simulink model "FFM_Punch"  (R2017a)
settings: Solver=ode3  StartTime=0.0  StopTime=timesteps  FixedStep=data.SIM.Ts  RelTol=1e-3  EnableMultiTasking=on
values from neighbouring files (symbols this model uses):
  data =     [dakota_config.mat]
  downshift_map = data.TCU.upshift.veh_spd_default    [Simulation_results.m]
  upshift_map = data.TCU.upshift.veh_spd_default    [Simulation_results.m]
undefined symbols (not defined in the file or in its folder): air_density, Cd, DiscIntNeverNeededParam, fr_crankshaft, fr_speed_values, g, i_FD, ICE, Low_Ratio, M_Eng_Max, M_Eng_Max_Max, M_Eng_Max_Rpm, mt2m_f, mu_Roll_C0, mu_Roll_C1, mu_Roll_C2, Mv, n_Idle_Eng, Overdrive_Ratio, Re, S_eff_drag, Ts
(part 5 of 15)

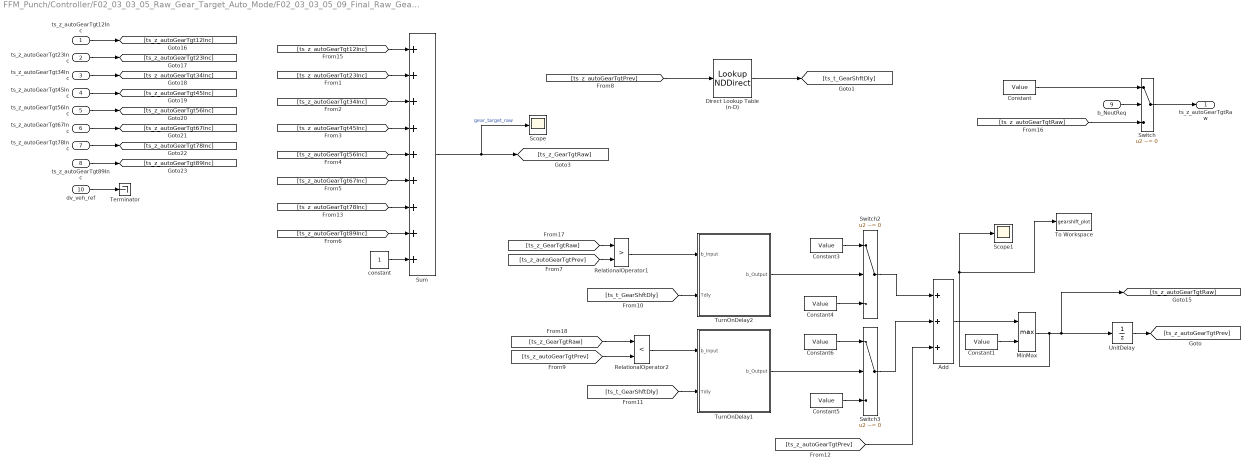
== system FFM_Punch/Controller/F02_03_03_05_Raw_Gear_Target_Auto_Mode/F02_03_03_05_09_Final_Raw_Gear_Target_Auto_Mode ==
  ts_z_autoGearTgt12Inc : Inport
  ts_z_autoGearTgt23Inc : Inport  Port=2
  ts_z_autoGearTgt34Inc : Inport  Port=3
  ts_z_autoGearTgt45Inc : Inport  Port=4
  ts_z_autoGearTgt56Inc : Inport  Port=5
  ts_z_autoGearTgt67Inc : Inport  Port=6
  ts_z_autoGearTgt78Inc : Inport  Port=7
  ts_z_autoGearTgt89Inc : Inport  Port=8
  b_NeutReq : Inport  Port=9
  dv_veh_ref : Inport  Tag=Controls_Lib  Description=Inp  Port=10  Interpolate=off
  Add : Sum  Inputs=+++
  Constant : Constant  Tag=Controls_Lib  Description=constant  Value=Value  OutMin=OutMin  OutMax=OutMax  OutDataTypeStr=int8  SampleTime=SampleTime  FramePeriod=FramePeriod  mask(Constant){Value=0, VectorParams1D=on, SampleTime=-1, FramePeriod=inf, OutMin=[], OutMax=[], OutDataTypeStr=int8, LockScale=off}
      mask prompts: Value "Simulink:blkprm_prompts:ConstConstValue"; VectorParams1D "Simulink:blkprm_prompts:AllSrcsVector1D"; SampleTime "Simulink:blkprm_prompts:AllSrcBlksSampleTime"; FramePeriod "Simulink:blkprm_prompts:AllSrcBlksFramePeriod"; OutMin "Simulink:blkprm_prompts:OutputDesignMin"; OutMax "Simulink:blkprm_prompts:OutputDesignMax"; OutDataTypeStr "Simulink:blkprm_prompts:OUTPUT_UNIFIEDDATATYPE"; LockScale "Simulink:blkprm_prompts:LockScale"
      mask help: Output the constant specified by the 'Constant value' parameter.
      mask Help: web([fileparts(which('Lib_built')) filesep 'hlp' filesep 'lib_constant' '.html'], '-helpbrowser')
      mask TypeOptions Value: Value
      mask TypeOptions VectorParams1D: VectorParams1D
      mask TypeOptions SampleTime: SampleTime
      mask TypeOptions FramePeriod: FramePeriod
      mask TypeOptions OutMin: OutMin
      mask TypeOptions OutMax: OutMax
      mask TypeOptions OutDataTypeStr: OutDataTypeStr
      mask TypeOptions LockScale: LockScale
      mask DialogControl ParameterTabVar0 Prompt: Main
      mask Display: disp(get_param(gcb,'Value'))
  Constant1 : Constant  Tag=Controls_Lib  Description=constant  Value=Value  OutMin=OutMin  OutMax=OutMax  OutDataTypeStr=int8  SampleTime=SampleTime  FramePeriod=FramePeriod  mask(Constant){Value=1, VectorParams1D=on, SampleTime=-1, FramePeriod=inf, OutMin=[], OutMax=[], OutDataTypeStr=int8, LockScale=off}
      mask prompts: Value "Simulink:blkprm_prompts:ConstConstValue"; VectorParams1D "Simulink:blkprm_prompts:AllSrcsVector1D"; SampleTime "Simulink:blkprm_prompts:AllSrcBlksSampleTime"; FramePeriod "Simulink:blkprm_prompts:AllSrcBlksFramePeriod"; OutMin "Simulink:blkprm_prompts:OutputDesignMin"; OutMax "Simulink:blkprm_prompts:OutputDesignMax"; OutDataTypeStr "Simulink:blkprm_prompts:OUTPUT_UNIFIEDDATATYPE"; LockScale "Simulink:blkprm_prompts:LockScale"
      mask help: Output the constant specified by the 'Constant value' parameter.
      mask Help: web([fileparts(which('Lib_built')) filesep 'hlp' filesep 'lib_constant' '.html'], '-helpbrowser')
      mask TypeOptions Value: Value
      mask TypeOptions VectorParams1D: VectorParams1D
      mask TypeOptions SampleTime: SampleTime
      mask TypeOptions FramePeriod: FramePeriod
      mask TypeOptions OutMin: OutMin
      mask TypeOptions OutMax: OutMax
      mask TypeOptions OutDataTypeStr: OutDataTypeStr
      mask TypeOptions LockScale: LockScale
      mask DialogControl ParameterTabVar0 Prompt: Main
      mask Display: disp(get_param(gcb,'Value'))
  Constant3 : Constant  Tag=Controls_Lib  Description=constant  Value=Value  OutMin=OutMin  OutMax=OutMax  OutDataTypeStr=int8  SampleTime=SampleTime  FramePeriod=FramePeriod  mask(Constant){Value=1, VectorParams1D=on, SampleTime=-1, FramePeriod=inf, OutMin=[], OutMax=[], OutDataTypeStr=int8, LockScale=off}
      mask prompts: Value "Simulink:blkprm_prompts:ConstConstValue"; VectorParams1D "Simulink:blkprm_prompts:AllSrcsVector1D"; SampleTime "Simulink:blkprm_prompts:AllSrcBlksSampleTime"; FramePeriod "Simulink:blkprm_prompts:AllSrcBlksFramePeriod"; OutMin "Simulink:blkprm_prompts:OutputDesignMin"; OutMax "Simulink:blkprm_prompts:OutputDesignMax"; OutDataTypeStr "Simulink:blkprm_prompts:OUTPUT_UNIFIEDDATATYPE"; LockScale "Simulink:blkprm_prompts:LockScale"
      mask help: Output the constant specified by the 'Constant value' parameter.
      mask Help: web([fileparts(which('Lib_built')) filesep 'hlp' filesep 'lib_constant' '.html'], '-helpbrowser')
      mask TypeOptions Value: Value
      mask TypeOptions VectorParams1D: VectorParams1D
      mask TypeOptions SampleTime: SampleTime
      mask TypeOptions FramePeriod: FramePeriod
      mask TypeOptions OutMin: OutMin
      mask TypeOptions OutMax: OutMax
      mask TypeOptions OutDataTypeStr: OutDataTypeStr
      mask TypeOptions LockScale: LockScale
      mask DialogControl ParameterTabVar0 Prompt: Main
      mask Display: disp(get_param(gcb,'Value'))
  Constant4 : Constant  Tag=Controls_Lib  Description=constant  Value=Value  OutMin=OutMin  OutMax=OutMax  OutDataTypeStr=int8  SampleTime=SampleTime  FramePeriod=FramePeriod  mask(Constant){Value=0, VectorParams1D=on, SampleTime=-1, FramePeriod=inf, OutMin=[], OutMax=[], OutDataTypeStr=int8, LockScale=off}
      mask prompts: Value "Simulink:blkprm_prompts:ConstConstValue"; VectorParams1D "Simulink:blkprm_prompts:AllSrcsVector1D"; SampleTime "Simulink:blkprm_prompts:AllSrcBlksSampleTime"; FramePeriod "Simulink:blkprm_prompts:AllSrcBlksFramePeriod"; OutMin "Simulink:blkprm_prompts:OutputDesignMin"; OutMax "Simulink:blkprm_prompts:OutputDesignMax"; OutDataTypeStr "Simulink:blkprm_prompts:OUTPUT_UNIFIEDDATATYPE"; LockScale "Simulink:blkprm_prompts:LockScale"
      mask help: Output the constant specified by the 'Constant value' parameter.
      mask Help: web([fileparts(which('Lib_built')) filesep 'hlp' filesep 'lib_constant' '.html'], '-helpbrowser')
      mask TypeOptions Value: Value
      mask TypeOptions VectorParams1D: VectorParams1D
      mask TypeOptions SampleTime: SampleTime
      mask TypeOptions FramePeriod: FramePeriod
      mask TypeOptions OutMin: OutMin
      mask TypeOptions OutMax: OutMax
      mask TypeOptions OutDataTypeStr: OutDataTypeStr
      mask TypeOptions LockScale: LockScale
      mask DialogControl ParameterTabVar0 Prompt: Main
      mask Display: disp(get_param(gcb,'Value'))
  Constant5 : Constant  Tag=Controls_Lib  Description=constant  Value=Value  OutMin=OutMin  OutMax=OutMax  OutDataTypeStr=int8  SampleTime=SampleTime  FramePeriod=FramePeriod  mask(Constant){Value=0, VectorParams1D=on, SampleTime=-1, FramePeriod=inf, OutMin=[], OutMax=[], OutDataTypeStr=int8, LockScale=off}
      mask prompts: Value "Simulink:blkprm_prompts:ConstConstValue"; VectorParams1D "Simulink:blkprm_prompts:AllSrcsVector1D"; SampleTime "Simulink:blkprm_prompts:AllSrcBlksSampleTime"; FramePeriod "Simulink:blkprm_prompts:AllSrcBlksFramePeriod"; OutMin "Simulink:blkprm_prompts:OutputDesignMin"; OutMax "Simulink:blkprm_prompts:OutputDesignMax"; OutDataTypeStr "Simulink:blkprm_prompts:OUTPUT_UNIFIEDDATATYPE"; LockScale "Simulink:blkprm_prompts:LockScale"
      mask help: Output the constant specified by the 'Constant value' parameter.
      mask Help: web([fileparts(which('Lib_built')) filesep 'hlp' filesep 'lib_constant' '.html'], '-helpbrowser')
      mask TypeOptions Value: Value
      mask TypeOptions VectorParams1D: VectorParams1D
      mask TypeOptions SampleTime: SampleTime
      mask TypeOptions FramePeriod: FramePeriod
      mask TypeOptions OutMin: OutMin
      mask TypeOptions OutMax: OutMax
      mask TypeOptions OutDataTypeStr: OutDataTypeStr
      mask TypeOptions LockScale: LockScale
      mask DialogControl ParameterTabVar0 Prompt: Main
      mask Display: disp(get_param(gcb,'Value'))
  Constant6 : Constant  Tag=Controls_Lib  Description=constant  Value=Value  OutMin=OutMin  OutMax=OutMax  OutDataTypeStr=int8  SampleTime=SampleTime  FramePeriod=FramePeriod  mask(Constant){Value=-1, VectorParams1D=on, SampleTime=-1, FramePeriod=inf, OutMin=[], OutMax=[], OutDataTypeStr=int8, LockScale=off}
      mask prompts: Value "Simulink:blkprm_prompts:ConstConstValue"; VectorParams1D "Simulink:blkprm_prompts:AllSrcsVector1D"; SampleTime "Simulink:blkprm_prompts:AllSrcBlksSampleTime"; FramePeriod "Simulink:blkprm_prompts:AllSrcBlksFramePeriod"; OutMin "Simulink:blkprm_prompts:OutputDesignMin"; OutMax "Simulink:blkprm_prompts:OutputDesignMax"; OutDataTypeStr "Simulink:blkprm_prompts:OUTPUT_UNIFIEDDATATYPE"; LockScale "Simulink:blkprm_prompts:LockScale"
      mask help: Output the constant specified by the 'Constant value' parameter.
      mask Help: web([fileparts(which('Lib_built')) filesep 'hlp' filesep 'lib_constant' '.html'], '-helpbrowser')
      mask TypeOptions Value: Value
      mask TypeOptions VectorParams1D: VectorParams1D
      mask TypeOptions SampleTime: SampleTime
      mask TypeOptions FramePeriod: FramePeriod
      mask TypeOptions OutMin: OutMin
      mask TypeOptions OutMax: OutMax
      mask TypeOptions OutDataTypeStr: OutDataTypeStr
      mask TypeOptions LockScale: LockScale
      mask DialogControl ParameterTabVar0 Prompt: Main
      mask Display: disp(get_param(gcb,'Value'))
  Direct Lookup Table (n-D) : LookupNDDirect  NumberOfTableDimensions=1  Table=data.TCU.gearShiftDelay  DiagnosticForOutOfRangeInput=None  TableDataTypeStr=single
  MinMax : MinMax  Function=max  Inputs=2
  RelationalOperator1 : RelationalOperator  Tag=Controls_Lib  Description=RelationalOperator  Operator=>  OutDataTypeStr=boolean  SampleTime=SampleTime  RndMeth=Nearest  InputSameDT=on  mask(Relational operator){Operator=>, ZeroCross=on, SampleTime=-1, InputSameDT=on, OutDataTypeStr=boolean}
      mask prompts: Operator "Relational operator:"; ZeroCross "Enable zero-crossing detection"; SampleTime "Sample time (-1 for inherited):"; InputSameDT "Require all inputs to have the same data type"; OutDataTypeStr "Output data type:"
      mask help: Applies the selected relational operator to the inputs and outputs the result. The top (or left) input corresponds to the first operand.
      mask Help: web([fileparts(which('Lib_built')) filesep 'hlp' filesep 'lib_Relational' '.html'], '-helpbrowser')
      mask TypeOptions Operator: Operator
      mask TypeOptions ZeroCross: ZeroCross
      mask TypeOptions SampleTime: SampleTime
      mask TypeOptions InputSameDT: InputSameDT
      mask TypeOptions OutDataTypeStr: OutDataTypeStr
  RelationalOperator2 : RelationalOperator  Tag=Controls_Lib  Description=RelationalOperator  Operator=<  OutDataTypeStr=boolean  SampleTime=SampleTime  RndMeth=Nearest  InputSameDT=on  mask(Relational operator){Operator=<, ZeroCross=on, SampleTime=-1, InputSameDT=on, OutDataTypeStr=boolean}
      mask prompts: Operator "Relational operator:"; ZeroCross "Enable zero-crossing detection"; SampleTime "Sample time (-1 for inherited):"; InputSameDT "Require all inputs to have the same data type"; OutDataTypeStr "Output data type:"
      mask help: Applies the selected relational operator to the inputs and outputs the result. The top (or left) input corresponds to the first operand.
      mask Help: web([fileparts(which('Lib_built')) filesep 'hlp' filesep 'lib_Relational' '.html'], '-helpbrowser')
      mask TypeOptions Operator: Operator
      mask TypeOptions ZeroCross: ZeroCross
      mask TypeOptions SampleTime: SampleTime
      mask TypeOptions InputSameDT: InputSameDT
      mask TypeOptions OutDataTypeStr: OutDataTypeStr
  Scope : Scope
  Scope1 : Scope
  Sum : Sum  Inputs=9  RndMeth=Zero  SaturateOnIntegerOverflow=on  InputSameDT=on  OutDataTypeStr=Inherit: Same as first input
  Switch : Switch  Tag=Controls_Lib  Description=Switch  Criteria=u2 ~= 0  Threshold=Threshold  OutMin=OutMin  OutMax=OutMax  OutDataTypeStr=Inherit: Inherit via back propagation  RndMeth=Zero  ZeroCross=off  SampleTime=SampleTime  InputSameDT=on  mask(Switch){Criteria=u2 ~= 0, Threshold=0.5, ZeroCross=off, SampleTime=-1, InputSameDT=on, OutMin=[], OutMax=[], OutDataTypeStr=Inherit: Inherit via back propagation, LockScale=off, RndMeth=Zero, SaturateOnIntegerOverflow=off, AllowDiffInputSizes=off}
      mask prompts: Criteria "Criteria for passing first input:"; ZeroCross "Enable zero-crossing detection"; SampleTime "Sample time (-1 for inherited):"; InputSameDT "Require all data port inputs to have the same data type"; OutMin "Output minimum:"; OutMax "Output maximum:"; OutDataTypeStr "Output data type:"; LockScale "Lock output data type setting against changes by the fixed-point tools"; RndMeth "Integer rounding mode:"; SaturateOnIntegerOverflow "Saturate on integer overflow"; AllowDiffInputSizes "Allow different data input sizes (Results in variable-size output signal)"
      mask help:
      | Pass through input 1 when input 2 is not equal to 0. Otherwise, pass through input 3.  The inputs are numbered top to bottom (or left to right). The input 1 pass-through criteria are input 2 not equal to 0;
      | The first and third input ports are data ports, and the second input port is the control port. The control port signal should always be a boolean signal.
      mask Help: web([fileparts(which('Lib_built')) filesep 'hlp' filesep 'lib_Switch' '.html'], '-helpbrowser')
      mask TypeOptions Criteria: Criteria
      mask TypeOptions Threshold: Threshold
      mask TypeOptions ZeroCross: ZeroCross
      mask TypeOptions SampleTime: SampleTime
      mask TypeOptions InputSameDT: InputSameDT
      mask TypeOptions OutMin: OutMin
      mask TypeOptions OutMax: OutMax
      mask TypeOptions OutDataTypeStr: OutDataTypeStr
      mask TypeOptions LockScale: LockScale
      mask TypeOptions RndMeth: RndMeth
      mask TypeOptions SaturateOnIntegerOverflow: SaturateOnIntegerOverflow
      mask TypeOptions AllowDiffInputSizes: AllowDiffInputSizes
  Switch2 : Switch  Tag=Controls_Lib  Description=Switch  Criteria=u2 ~= 0  Threshold=Threshold  OutMin=OutMin  OutMax=OutMax  OutDataTypeStr=Inherit: Inherit via back propagation  RndMeth=Zero  ZeroCross=off  SampleTime=SampleTime  InputSameDT=on  mask(Switch){Criteria=u2 ~= 0, Threshold=0.5, ZeroCross=off, SampleTime=-1, InputSameDT=on, OutMin=[], OutMax=[], OutDataTypeStr=Inherit: Inherit via back propagation, LockScale=off, RndMeth=Zero, SaturateOnIntegerOverflow=off, AllowDiffInputSizes=off}
      mask prompts: Criteria "Criteria for passing first input:"; ZeroCross "Enable zero-crossing detection"; SampleTime "Sample time (-1 for inherited):"; InputSameDT "Require all data port inputs to have the same data type"; OutMin "Output minimum:"; OutMax "Output maximum:"; OutDataTypeStr "Output data type:"; LockScale "Lock output data type setting against changes by the fixed-point tools"; RndMeth "Integer rounding mode:"; SaturateOnIntegerOverflow "Saturate on integer overflow"; AllowDiffInputSizes "Allow different data input sizes (Results in variable-size output signal)"
      mask help:
      | Pass through input 1 when input 2 is not equal to 0. Otherwise, pass through input 3.  The inputs are numbered top to bottom (or left to right). The input 1 pass-through criteria are input 2 not equal to 0;
      | The first and third input ports are data ports, and the second input port is the control port. The control port signal should always be a boolean signal.
      mask Help: web([fileparts(which('Lib_built')) filesep 'hlp' filesep 'lib_Switch' '.html'], '-helpbrowser')
      mask TypeOptions Criteria: Criteria
      mask TypeOptions Threshold: Threshold
      mask TypeOptions ZeroCross: ZeroCross
      mask TypeOptions SampleTime: SampleTime
      mask TypeOptions InputSameDT: InputSameDT
      mask TypeOptions OutMin: OutMin
      mask TypeOptions OutMax: OutMax
      mask TypeOptions OutDataTypeStr: OutDataTypeStr
      mask TypeOptions LockScale: LockScale
      mask TypeOptions RndMeth: RndMeth
      mask TypeOptions SaturateOnIntegerOverflow: SaturateOnIntegerOverflow
      mask TypeOptions AllowDiffInputSizes: AllowDiffInputSizes
  Switch3 : Switch  Tag=Controls_Lib  Description=Switch  Criteria=u2 ~= 0  Threshold=Threshold  OutMin=OutMin  OutMax=OutMax  OutDataTypeStr=Inherit: Inherit via back propagation  RndMeth=Zero  ZeroCross=off  SampleTime=SampleTime  InputSameDT=on  mask(Switch){Criteria=u2 ~= 0, Threshold=0.5, ZeroCross=off, SampleTime=-1, InputSameDT=on, OutMin=[], OutMax=[], OutDataTypeStr=Inherit: Inherit via back propagation, LockScale=off, RndMeth=Zero, SaturateOnIntegerOverflow=off, AllowDiffInputSizes=off}
      mask prompts: Criteria "Criteria for passing first input:"; ZeroCross "Enable zero-crossing detection"; SampleTime "Sample time (-1 for inherited):"; InputSameDT "Require all data port inputs to have the same data type"; OutMin "Output minimum:"; OutMax "Output maximum:"; OutDataTypeStr "Output data type:"; LockScale "Lock output data type setting against changes by the fixed-point tools"; RndMeth "Integer rounding mode:"; SaturateOnIntegerOverflow "Saturate on integer overflow"; AllowDiffInputSizes "Allow different data input sizes (Results in variable-size output signal)"
      mask help:
      | Pass through input 1 when input 2 is not equal to 0. Otherwise, pass through input 3.  The inputs are numbered top to bottom (or left to right). The input 1 pass-through criteria are input 2 not equal to 0;
      | The first and third input ports are data ports, and the second input port is the control port. The control port signal should always be a boolean signal.
      mask Help: web([fileparts(which('Lib_built')) filesep 'hlp' filesep 'lib_Switch' '.html'], '-helpbrowser')
      mask TypeOptions Criteria: Criteria
      mask TypeOptions Threshold: Threshold
      mask TypeOptions ZeroCross: ZeroCross
      mask TypeOptions SampleTime: SampleTime
      mask TypeOptions InputSameDT: InputSameDT
      mask TypeOptions OutMin: OutMin
      mask TypeOptions OutMax: OutMax
      mask TypeOptions OutDataTypeStr: OutDataTypeStr
      mask TypeOptions LockScale: LockScale
      mask TypeOptions RndMeth: RndMeth
      mask TypeOptions SaturateOnIntegerOverflow: SaturateOnIntegerOverflow
      mask TypeOptions AllowDiffInputSizes: AllowDiffInputSizes
  Terminator : Terminator
  To Workspace : ToWorkspace  VariableName=gearshift_plot  SampleTime=-1
  TurnOnDelay1 : Subsystem  Tag=Controls_Lib  Description=Turn_on_off_delay  mask(Turn ON Delay){}
      mask help:
      | Turn ON Delay block introduces the delay(Tdly) in the Input signal.The Input signal is delayed by Tdly when rising edge in the Input signal is detected.The Output is set to true  if Input is true for 'Tdly'.
      |
      | Inputs:
      | b_Input : Input coming to the Turn On Delay block
      | Tdly      : Time Delay defined externally by user
      |
      | Output:
      | Output : Output of the Turn On Delay block
      |
      | Notes:
      | 1. Input 'Tdly' must always be positive non-zero number and must be a multiple of the fundamental sample time of the block.
      | 2. Input to this block should always be boolean
      mask Help: web([fileparts(which('Lib_math_logic')) filesep 'hlp' filesep 'lib_TurnOnOffDelay.html'], '-helpbrowser')
      mask Display:
      | plot([0.9 0.65 0.65 0.1],[0.75 0.75 0.1 0.1]);
      | plot([0.9 0.35 0.35 0.1],[0.85 0.85 0.2 0.2]);
      | plot([0.35 0.65],[0.5 0.5]);
      | text(0.23,0.95,'Turn-on Delay');
      | text(0.43,0.55,'Tdly');
      | plot([0.4 0.35 0.4],[0.48 0.5 0.52]);
      | plot([0.6 0.65 0.6],[0.48 0.5 0.52]);
  TurnOnDelay2 : Subsystem  Tag=Controls_Lib  Description=Turn_on_off_delay  mask(Turn ON Delay){}
      mask help:
      | Turn ON Delay block introduces the delay(Tdly) in the Input signal.The Input signal is delayed by Tdly when rising edge in the Input signal is detected.The Output is set to true  if Input is true for 'Tdly'.
      |
      | Inputs:
      | b_Input : Input coming to the Turn On Delay block
      | Tdly      : Time Delay defined externally by user
      |
      | Output:
      | Output : Output of the Turn On Delay block
      |
      | Notes:
      | 1. Input 'Tdly' must always be positive non-zero number and must be a multiple of the fundamental sample time of the block.
      | 2. Input to this block should always be boolean
      mask Help: web([fileparts(which('Lib_math_logic')) filesep 'hlp' filesep 'lib_TurnOnOffDelay.html'], '-helpbrowser')
      mask Display:
      | plot([0.9 0.65 0.65 0.1],[0.75 0.75 0.1 0.1]);
      | plot([0.9 0.35 0.35 0.1],[0.85 0.85 0.2 0.2]);
      | plot([0.35 0.65],[0.5 0.5]);
      | text(0.23,0.95,'Turn-on Delay');
      | text(0.43,0.55,'Tdly');
      | plot([0.4 0.35 0.4],[0.48 0.5 0.52]);
      | plot([0.6 0.65 0.6],[0.48 0.5 0.52]);
  UnitDelay : UnitDelay  Tag=Controls_Lib  Description=UnitDelay  InitialCondition=X0  SampleTime=SampleTime  mask(Unit delay){X0=1, InputProcessing=Elements as channels (sample based), SampleTime=-1, StateIdentifier=, StateMustResolveToSignalObject=off, RTWStateStorageClass=Auto, RTWStateStorageTypeQualifier=}
      mask prompts: X0 "Initial conditions:"; InputProcessing "Input processing:"; SampleTime "Sample time (-1 for inherited):"; StateIdentifier "State name:"; StateMustResolveToSignalObject "State name must resolve to Simulink signal object"; RTWStateStorageClass "Code generation storage class:"; RTWStateStorageTypeQualifier "Code generation storage type qualifier:"
      mask help: Delays input signal by one sample period
      settings: AttributesFormatString=Init_con=%<X0>
      mask Help: web([fileparts(which('Lib_discrete')) filesep 'hlp' filesep 'lib_UnitDelay.html'], '-helpbrowser')
      mask TypeOptions X0: X0
      mask TypeOptions InputProcessing: InputProcessing
      mask TypeOptions SampleTime: SampleTime
      mask TypeOptions StateIdentifier: StateIdentifier
      mask TypeOptions StateMustResolveToSignalObject: StateMustResolveToSignalObject
      mask TypeOptions RTWStateStorageClass: RTWStateStorageClass
      mask TypeOptions RTWStateStorageTypeQualifier: RTWStateStorageTypeQualifier
  constant : Constant  OutDataTypeStr=int8
  ts_z_autoGearTgtRaw : Outport
  wires:
  ts_z_autoGearTgt89Inc/1 -> [ts_z_autoGearTgt89Inc]
  ts_z_autoGearTgt78Inc/1 -> [ts_z_autoGearTgt78Inc]
  [ts_z_autoGearTgt89Inc] -> Sum/8
  [ts_z_autoGearTgt78Inc] -> Sum/7
  constant/1 -> Sum/9
  [ts_z_autoGearTgt12Inc] -> Sum/1
  [ts_z_autoGearTgt23Inc] -> Sum/2
  [ts_z_autoGearTgt34Inc] -> Sum/3
  [ts_z_autoGearTgt45Inc] -> Sum/4
  [ts_z_autoGearTgt56Inc] -> Sum/5
  [ts_z_autoGearTgt67Inc] -> Sum/6
  [ts_z_autoGearTgtRaw] -> Switch/3
  ts_z_autoGearTgt12Inc/1 -> [ts_z_autoGearTgt12Inc]
  ts_z_autoGearTgt23Inc/1 -> [ts_z_autoGearTgt23Inc]
  ts_z_autoGearTgt34Inc/1 -> [ts_z_autoGearTgt34Inc]
  ts_z_autoGearTgt45Inc/1 -> [ts_z_autoGearTgt45Inc]
  ts_z_autoGearTgt56Inc/1 -> [ts_z_autoGearTgt56Inc]
  ts_z_autoGearTgt67Inc/1 -> [ts_z_autoGearTgt67Inc]
  b_NeutReq/1 -> Switch/2
  Switch/1 -> ts_z_autoGearTgtRaw/1
  Constant/1 -> Switch/1
  Sum/1 -> Scope/1, [ts_z_GearTgtRaw]  "gear_target_raw"
  [ts_z_autoGearTgtPrev] -> Direct Lookup Table (n-D)/1
  UnitDelay/1 -> [ts_z_autoGearTgtPrev]
  [ts_z_autoGearTgtPrev] -> RelationalOperator1/2
  [ts_z_autoGearTgtPrev] -> RelationalOperator2/2
  RelationalOperator1/1 -> TurnOnDelay2/1(b_Input)
  RelationalOperator2/1 -> TurnOnDelay1/1(b_Input)
  [ts_t_GearShftDly] -> TurnOnDelay1/2(Tdly)
  [ts_z_GearTgtRaw] -> RelationalOperator1/1
  [ts_z_GearTgtRaw] -> RelationalOperator2/1
  Direct Lookup Table (n-D)/1 -> [ts_t_GearShftDly]
  [ts_t_GearShftDly] -> TurnOnDelay2/2(Tdly)
  Constant3/1 -> Switch2/1
  Constant4/1 -> Switch2/3
  Constant5/1 -> Switch3/3
  TurnOnDelay1/1(b_Output) -> Switch3/2
  Constant6/1 -> Switch3/1
  Switch2/1 -> Add/1
  Switch3/1 -> Add/2
  [ts_z_autoGearTgtPrev] -> Add/3
  dv_veh_ref/1 -> Terminator/1
  TurnOnDelay2/1(b_Output) -> Switch2/2
  Add/1 -> MinMax/1
  Constant1/1 -> MinMax/2
  MinMax/1 -> To Workspace/1, Scope1/1, UnitDelay/1, [ts_z_autoGearTgtRaw]

== system FFM_Punch/Driver Interface/Driver Mode_pedalbased/Driver PID Error Calculation and ffwd ==
  v_Ref : Inport
  v_Veh : Inport  Port=2
  F_load : Inport  Port=3
  dv_veh : Inport  Port=4
  r_Overall : Inport  Port=5
  M_eng_Max : Inport  Port=6
  Constant2 : Constant  Tag=Controls_Lib  Description=constant  Value=Value  OutMin=OutMin  OutMax=OutMax  OutDataTypeStr=Inherit: Inherit via back propagation  SampleTime=SampleTime  FramePeriod=FramePeriod  mask(Constant){Value=0, VectorParams1D=on, SampleTime=-1, FramePeriod=inf, OutMin=[], OutMax=[], OutDataTypeStr=Inherit: Inherit via back propagation, LockScale=off}
      mask prompts: Value "Simulink:blkprm_prompts:ConstConstValue"; VectorParams1D "Simulink:blkprm_prompts:AllSrcsVector1D"; SampleTime "Simulink:blkprm_prompts:AllSrcBlksSampleTime"; FramePeriod "Simulink:blkprm_prompts:AllSrcBlksFramePeriod"; OutMin "Simulink:blkprm_prompts:OutputDesignMin"; OutMax "Simulink:blkprm_prompts:OutputDesignMax"; OutDataTypeStr "Simulink:blkprm_prompts:OUTPUT_UNIFIEDDATATYPE"; LockScale "Simulink:blkprm_prompts:LockScale"
      mask help: Output the constant specified by the 'Constant value' parameter.
      mask Help: web([fileparts(which('Lib_built')) filesep 'hlp' filesep 'lib_constant' '.html'], '-helpbrowser')
      mask TypeOptions Value: Value
      mask TypeOptions VectorParams1D: VectorParams1D
      mask TypeOptions SampleTime: SampleTime
      mask TypeOptions FramePeriod: FramePeriod
      mask TypeOptions OutMin: OutMin
      mask TypeOptions OutMax: OutMax
      mask TypeOptions OutDataTypeStr: OutDataTypeStr
      mask TypeOptions LockScale: LockScale
      mask DialogControl ParameterTabVar0 Prompt: Main
      mask Display: disp(get_param(gcb,'Value'))
  Constant3 : Constant  Tag=Controls_Lib  Description=constant  Value=Value  OutMin=OutMin  OutMax=OutMax  OutDataTypeStr=Inherit: Inherit via back propagation  SampleTime=SampleTime  FramePeriod=FramePeriod  mask(Constant){Value=1, VectorParams1D=on, SampleTime=-1, FramePeriod=inf, OutMin=[], OutMax=[], OutDataTypeStr=Inherit: Inherit via back propagation, LockScale=off}
      mask prompts: Value "Simulink:blkprm_prompts:ConstConstValue"; VectorParams1D "Simulink:blkprm_prompts:AllSrcsVector1D"; SampleTime "Simulink:blkprm_prompts:AllSrcBlksSampleTime"; FramePeriod "Simulink:blkprm_prompts:AllSrcBlksFramePeriod"; OutMin "Simulink:blkprm_prompts:OutputDesignMin"; OutMax "Simulink:blkprm_prompts:OutputDesignMax"; OutDataTypeStr "Simulink:blkprm_prompts:OUTPUT_UNIFIEDDATATYPE"; LockScale "Simulink:blkprm_prompts:LockScale"
      mask help: Output the constant specified by the 'Constant value' parameter.
      mask Help: web([fileparts(which('Lib_built')) filesep 'hlp' filesep 'lib_constant' '.html'], '-helpbrowser')
      mask TypeOptions Value: Value
      mask TypeOptions VectorParams1D: VectorParams1D
      mask TypeOptions SampleTime: SampleTime
      mask TypeOptions FramePeriod: FramePeriod
      mask TypeOptions OutMin: OutMin
      mask TypeOptions OutMax: OutMax
      mask TypeOptions OutDataTypeStr: OutDataTypeStr
      mask TypeOptions LockScale: LockScale
      mask DialogControl ParameterTabVar0 Prompt: Main
      mask Display: disp(get_param(gcb,'Value'))
  Constant5 : Constant  Tag=Controls_Lib  Description=constant  Value=Value  OutMin=OutMin  OutMax=OutMax  OutDataTypeStr=Inherit: Inherit via back propagation  SampleTime=SampleTime  FramePeriod=FramePeriod  mask(Constant){Value=0, VectorParams1D=on, SampleTime=-1, FramePeriod=inf, OutMin=[], OutMax=[], OutDataTypeStr=Inherit: Inherit via back propagation, LockScale=off}
      mask prompts: Value "Simulink:blkprm_prompts:ConstConstValue"; VectorParams1D "Simulink:blkprm_prompts:AllSrcsVector1D"; SampleTime "Simulink:blkprm_prompts:AllSrcBlksSampleTime"; FramePeriod "Simulink:blkprm_prompts:AllSrcBlksFramePeriod"; OutMin "Simulink:blkprm_prompts:OutputDesignMin"; OutMax "Simulink:blkprm_prompts:OutputDesignMax"; OutDataTypeStr "Simulink:blkprm_prompts:OUTPUT_UNIFIEDDATATYPE"; LockScale "Simulink:blkprm_prompts:LockScale"
      mask help: Output the constant specified by the 'Constant value' parameter.
      mask Help: web([fileparts(which('Lib_built')) filesep 'hlp' filesep 'lib_constant' '.html'], '-helpbrowser')
      mask TypeOptions Value: Value
      mask TypeOptions VectorParams1D: VectorParams1D
      mask TypeOptions SampleTime: SampleTime
      mask TypeOptions FramePeriod: FramePeriod
      mask TypeOptions OutMin: OutMin
      mask TypeOptions OutMax: OutMax
      mask TypeOptions OutDataTypeStr: OutDataTypeStr
      mask TypeOptions LockScale: LockScale
      mask DialogControl ParameterTabVar0 Prompt: Main
      mask Display: disp(get_param(gcb,'Value'))
  Convert : DataTypeConversion  Tag=Controls_Lib  Description=Convert  OutMin=OutMin  OutMax=OutMax  RndMeth=Round  SampleTime=SampleTime  SaturateOnIntegerOverflow=on  mask(Datatype conversion){ConvertRealWorld=Real World Value (RWV), SampleTime=-1, OutMin=[], OutMax=[], OutDataTypeStr=Inherit: Inherit via back propagation, LockScale=off, RndMeth=Round, SaturateOnIntegerOverflow=on}
      mask prompts: ConvertRealWorld "Input and output to have equal:"; SampleTime "Sample time (-1 for inherited):"; OutMin "Output minimum:"; OutMax "Output maximum:"; OutDataTypeStr "Output data type:"; LockScale "Lock output data type setting against changes by the fixed-point tools"; RndMeth "Integer rounding mode:"; SaturateOnIntegerOverflow "Saturate on integer overflow"
      mask help: Convert the input to the data type and scaling of the output.
      mask Help: web([fileparts(which('Lib_built')) filesep 'hlp' filesep 'lib_DataTypeConv' '.html'], '-helpbrowser')
      mask TypeOptions ConvertRealWorld: ConvertRealWorld
      mask TypeOptions SampleTime: SampleTime
      mask TypeOptions OutMin: OutMin
      mask TypeOptions OutMax: OutMax
      mask TypeOptions OutDataTypeStr: OutDataTypeStr
      mask TypeOptions LockScale: LockScale
      mask TypeOptions RndMeth: RndMeth
      mask TypeOptions SaturateOnIntegerOverflow: SaturateOnIntegerOverflow
  Convert1 : DataTypeConversion  Tag=Controls_Lib  Description=Convert  OutMin=OutMin  OutMax=OutMax  RndMeth=Round  SampleTime=SampleTime  SaturateOnIntegerOverflow=on  mask(Datatype conversion){ConvertRealWorld=Real World Value (RWV), SampleTime=-1, OutMin=[], OutMax=[], OutDataTypeStr=Inherit: Inherit via back propagation, LockScale=off, RndMeth=Round, SaturateOnIntegerOverflow=on}
      mask prompts: ConvertRealWorld "Input and output to have equal:"; SampleTime "Sample time (-1 for inherited):"; OutMin "Output minimum:"; OutMax "Output maximum:"; OutDataTypeStr "Output data type:"; LockScale "Lock output data type setting against changes by the fixed-point tools"; RndMeth "Integer rounding mode:"; SaturateOnIntegerOverflow "Saturate on integer overflow"
      mask help: Convert the input to the data type and scaling of the output.
      mask Help: web([fileparts(which('Lib_built')) filesep 'hlp' filesep 'lib_DataTypeConv' '.html'], '-helpbrowser')
      mask TypeOptions ConvertRealWorld: ConvertRealWorld
      mask TypeOptions SampleTime: SampleTime
      mask TypeOptions OutMin: OutMin
      mask TypeOptions OutMax: OutMax
      mask TypeOptions OutDataTypeStr: OutDataTypeStr
      mask TypeOptions LockScale: LockScale
      mask TypeOptions RndMeth: RndMeth
      mask TypeOptions SaturateOnIntegerOverflow: SaturateOnIntegerOverflow
  FirstOrderDerivative1 : Subsystem  Tag=Controls_Lib  Description=DiscreteDerivative  mask(Discrete Derivative Block){}
      mask help:
      | Computes the discrete derivative of the input signal as the rate of change of signal with respect to Sampling Time.
      |
      | Inputs:
      | Input         : Signal to be Filtered
      |
      |
      |
      | Outputs:
      | Output : Filter Output of the Discrete Derivative block
      mask Help: web([fileparts(which('Lib_discrete')) filesep 'hlp' filesep 'lib_DiscreteDerivative.html'], '-helpbrowser')
      mask Display: disp('Discrete\nDerivative');
  FirstOrderLPF1 : Subsystem  Tag=Controls_Lib  Description=FirstOrderLowPassFilter  RTWFcnName=Derivative_1_intial  mask(First Order Low Pass Filter){}
      mask help:
      | The First Order Low Pass Filter allows signals with a frequency lower than a certain cutoff frequency (fc) to pass through the block and attenuates signals with frequencies higher than the cutoff frequency (fc or wc).
      |
      | Inputs:
      | Input        : Signal to be Filtered
      | Tau          : Filter Time Constant (1/2*pi*fc) in Seconds defined externally
      |                  by user
      | b_Reset    : Initialization flag can be used for
      |                   controlling the filter initialization
      |                   with a non-zero initial condition “ResetValue”
      |                   When b_Reset == TRUE → Out(k)=ResetValue defined externally by
      |                   user
      | ResetValue : Filter Initial Condition defined externally by user
      |
      | Output :
      | Output : Filter Output
      |
      | Notes :
      | 1. Filter time constant should be selected such that the cut-off
      |     frequency (fc)is higher than the bandwidth of the control system.
      | 2. At First sample the b_Reset should be FALSE.
      settings: RTWFileNameOpts=Use function name
      mask Help: web([fileparts(which('Lib_discrete')) filesep 'hlp' filesep 'lib_FirstOrderLPF.html'], '-helpbrowser')
      mask Display: disp('First order\nLow Pass\nFilter');
  Gain2 : Gain  Gain=0.5  OutDataTypeStr=Inherit: Same as input
  Gain3 : Gain  Gain=1/3.6  OutDataTypeStr=Inherit: Same as input
  Inertia : Fcn  Expr=data.VEH.Mv*(1+data.VEH.eqv_inertia)*u
  Sum1 : Sum  Inputs=|+-
  Terminator : Terminator
  Terminator1 : Terminator
  Throttle_Pedal_Determination : Subsystem
  err_drv_PIDvehSpd : Outport
  throttle_ffwd : Outport  Port=2
  dv_veh_ref : Outport  Port=3
  wires:
  Convert1/1 -> [v_Ref]
  Convert/1 -> [v_Veh]
  v_Ref/1 -> Convert1/1
  v_Veh/1 -> Convert/1
  Throttle_Pedal_Determination/1(Perc_Throtlle_FFWD) -> throttle_ffwd/1
  [v_Veh] -> Sum1/2
  [v_Ref] -> Sum1/1
  dv_veh/1 -> Terminator1/1
  Gain3/1 -> Inertia/1
  F_load/1 -> Terminator/1
  Inertia/1 -> Gain2/1  "FFD_dyn"
  [v_Ref] -> FirstOrderDerivative1/1(Input)
  [dv_veh_ref] -> Gain3/1
  r_Overall/1 -> [r_Overall]
  Gain2/1 -> Throttle_Pedal_Determination/2(Mwheel_FFWD)
  [r_Overall] -> Throttle_Pedal_Determination/1(r_Overall)
  M_eng_Max/1 -> [M_eng_Max]
  [M_eng_Max] -> Throttle_Pedal_Determination/3(M_eng_Max)
  [dv_veh_ref] -> dv_veh_ref/1
  Sum1/1 -> err_drv_PIDvehSpd/1
  Constant3/1 -> FirstOrderLPF1/2(Tau)
  Constant2/1 -> FirstOrderLPF1/3(b_Reset)
  Constant5/1 -> FirstOrderLPF1/4(ResetValue)
  FirstOrderLPF1/1(Output) -> [dv_veh_ref]
  FirstOrderDerivative1/1(Output) -> FirstOrderLPF1/1(Input)  "dv_ref"
